simulink model "test_pmdc_speed_control"  (R2023a)
settings: Solver=FixedStepAuto  StartTime=0.0  StopTime=2  FixedStep=1e-5  RelTol=1e-3
values from neighbouring files (symbols this model uses):
  J = 0.05    [dcmotor_parameter.m]    (also in parabtl.m; pmdc_parameter.m = 0.00252; testpara.m = 0.00252)
  Ki = Kp/Ti    [parabtl.m]    (also in pmdc_parameter.m)
  Kiv = Kpv/Tiv    [parabtl.m]    (also in pmdc_parameter.m)
  Kp = (Ra*Ta*OmegaN)/(2*Zeta)    [parabtl.m]    (also in pmdc_parameter.m)
  Kpv = TMech/(2*Teq)    [parabtl.m]    (also in pmdc_parameter.m)
  KT = KE    (= 1.17113806452)    [dcmotor_parameter.m]    (also in parabtl.m; pmdc_parameter.m = 0.424975; testpara.m = 0.424975)
  La = 5.2e-3    (= 0.0052)    [dcmotor_parameter.m]    (also in parabtl.m; pmdc_parameter.m = 0.0017; testpara.m = 0.0017)
  Ra = 0.32    [dcmotor_parameter.m]    (also in parabtl.m; pmdc_parameter.m = 0.26; testpara.m = 0.26)
  Tfi = 1/(5*fsw)    (= 4e-05)    [parabtl.m]    (also in pmdc_parameter.m)
  Tfv = 5*Tfi    (= 0.0002)    [parabtl.m]    (also in pmdc_parameter.m)
  UaN = 400    [parabtl.m]    (also in pmdc_parameter.m = 140; testpara.m = 140)
libraries: spsMosfetLib x16, spsVoltageMeasurementLib x5, spsDCMachineLib x4, spsDCVoltageSourceLib x4, simulink x4, spsControlledVoltageSourceLib x1, sps_lib x1
settings Model: Creator=luand  LastModifiedBy=luand

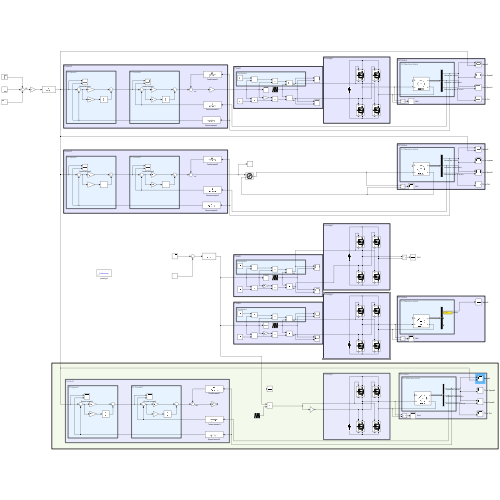
[thumbnail: Simulink's stored preview of the top-level diagram]
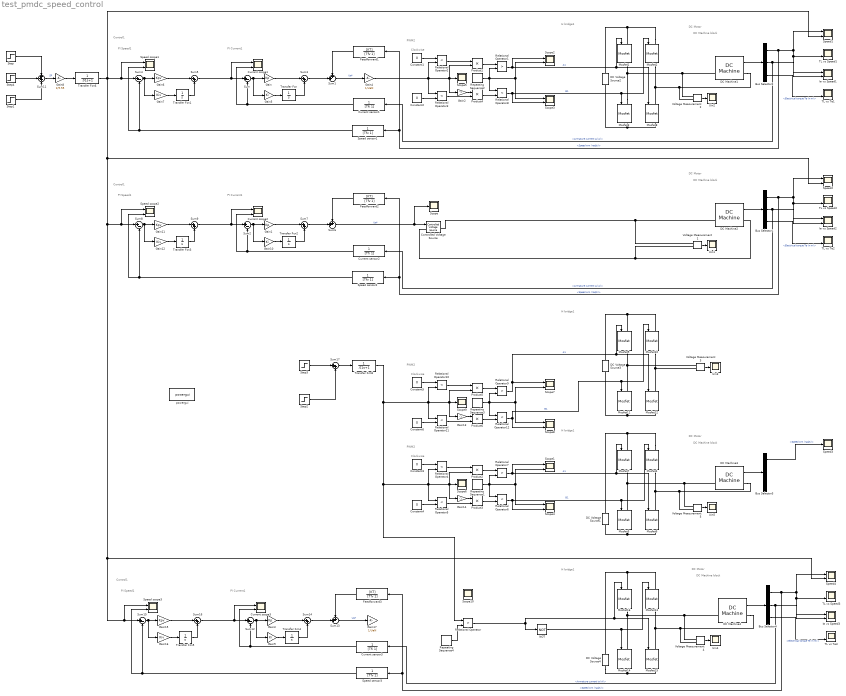
== system test_pmdc_speed_control ==
  note: PI Speed1
  note: PI Current1
  note: H bridge1
  note: PWM2
  note: Control1
  note: DC Motor
  note: DC Machine block
  note: Clockwise
  note: PI Speed1
  note: PI Current1
  note: Control1
  note: DC Motor
  note: DC Machine block
  note: H bridge1
  note: PWM2
  note: Clockwise
  note: H bridge1
  note: PWM2
  note: Clockwise
  note: DC Motor
  note: DC Machine block
  note: PI Speed1
  note: PI Current1
  note: Control1
  note: DC Motor
  note: DC Machine block
  note: H bridge1
  Bus Selector{1..4} (4 alike) : BusSelector  OutputSignals=Speed wm (rad/s),Armature current ia (A),Electrical torque Te (n m)
  Constant{1..6} (6 alike) : Constant  Value=0
  Controlled Voltage Source : spsControlledVoltageSourceLib/Controlled Voltage Source  Initialize=on  Source_Type=DC  Amplitude=0  Phase=0  Frequency=0  Measurements=None
  Current scope1 : Scope  NumInputPorts=2
  Current scope2 : Scope  NumInputPorts=2
  Current scope3 : Scope  NumInputPorts=2
  Current sensor1 : TransferFcn  Denominator=[Tfi 1]
  Current sensor2 : TransferFcn  Denominator=[Tfi 1]
  Current sensor3 : TransferFcn  Denominator=[Tfi 1]
  DC Machine{1..4} (4 alike) : spsDCMachineLib/DC Machine  PresetModel=No  MechanicalLoad=Torque TL  FieldType=Permanent magnet  ShowDetailedParameters=on  MeasurementBus=off  RLa=[ Ra La ]  RLf="[ 240  120]"  Laf=1.8  MachineConstant=Torque constant (N.m/A)  Ke=1.8  Kt=KT  J=J  Bm=0  Tf=0  w0=0  Ifinit=1  TsPowergui=0  TsBlock=-1
  DC Voltage Source{1..4} (4 alike) : spsDCVoltageSourceLib/DC Voltage Source  Amplitude=UaN  Measurements=None
  Feedforward1 : TransferFcn  Numerator=[KT]  Denominator=[Tfv 1]
  Feedforward2 : TransferFcn  Numerator=[KT]  Denominator=[Tfv 1]
  Feedforward3 : TransferFcn  Numerator=[KT]  Denominator=[Tfv 1]
  Gain : Gain  Gain=Kp
  Gain1 : Gain  Gain=Kp
  Gain10 : Gain  Gain=Ki
  Gain11 : Gain  Gain=Kpv
  Gain12 : Gain  Gain=Kiv
  Gain13 : Gain  Gain=-1
  Gain14 : Gain  Gain=-1
  Gain15 : Gain  Gain=Kpv
  Gain16 : Gain  Gain=Kiv
  Gain17 : Gain  Gain=1/UaN
  Gain2 : Gain  Gain=-1
  Gain3 : Gain  Gain=Kp
  Gain4 : Gain  Gain=1/UaN
  Gain5 : Gain  Gain=Ki
  Gain6 : Gain  Gain=Kpv
  Gain7 : Gain  Gain=Kiv
  Gain8 : Gain  Gain=1/9.55
  Gain9 : Gain  Gain=Ki
  Ia vs Speed1 : Scope  NumInputPorts=2
  Ia vs Speed2 : Scope  NumInputPorts=2
  Ia vs Speed3 : Scope  NumInputPorts=2
  Mosfet{1..3,8} (4 alike) : spsMosfetLib/Mosfet  Ron=0.1  Lon=0  Rd=0.01  Vfd=0  IC=0  Rs=1e5  Cs=inf  Measurements=on
  Mosfet{4..7,9..16} (12 alike) : spsMosfetLib/Mosfet  Ron=1e-3  Lon=0  Rd=0.01  Vfd=0  IC=0  Rs=1e5  Cs=inf  Measurements=on
  NOT : Logic  Operator=NOT  IconShape=distinctive  AllPortsSameDT=off  OutDataTypeStr=boolean
  Product{1..6} (6 alike) : Product
  Relational Operator{,1,7,9} (4 alike) : RelationalOperator  Operator=>  OutDataTypeStr=boolean  RndMeth=Simplest  InputSameDT=off
  Relational Operator{2..6,8,10..12} (9 alike) : RelationalOperator  Operator=<  OutDataTypeStr=boolean  RndMeth=Simplest  InputSameDT=off
  Repeating Sequence1 : simulink/Sources/Repeating Sequence  rep_seq_t=[0 1e-3]  rep_seq_y=[0 1]
  Repeating Sequence2 : simulink/Sources/Repeating Sequence  rep_seq_t=[0 1e-3]  rep_seq_y=[0 1]
  Repeating Sequence3 : simulink/Sources/Repeating Sequence  rep_seq_t=[0 1e-3]  rep_seq_y=[0 1]
  Repeating Sequence4 : simulink/Sources/Repeating Sequence  rep_seq_t=[0 5e-4 1e-3]  rep_seq_y=[-1 1 -1]
  Scope{,5..6,9..10} (5 alike) : Scope
  Scope{1..4,7..8} (6 alike) : Scope  NumInputPorts=2
  Speed scope1 : Scope  NumInputPorts=2
  Speed scope2 : Scope  NumInputPorts=2
  Speed scope3 : Scope  NumInputPorts=2
  Speed sensor1 : TransferFcn  Denominator=[Tfv 1]
  Speed sensor2 : TransferFcn  Denominator=[Tfv 1]
  Speed sensor3 : TransferFcn  Denominator=[Tfv 1]
  Speed1 : Scope  NumInputPorts=2
  Speed2 : Scope  NumInputPorts=2
  Speed3 : Scope
  Speed4 : Scope  NumInputPorts=2
  Step : Step  Time=0  After=3000  SampleTime=0
  Step1 : Step  Time=2  After=-1500  SampleTime=0
  Step2 : Step  After=-1  SampleTime=0
  Step3 : Step  Time=0  After=.5  SampleTime=0
  Step4 : Step  After=-1500  SampleTime=0
  Sum{,2,4,8,12,15} (6 alike) : Sum  Inputs=|+-
  Sum1 : Sum  Inputs=++|
  Sum11 : Sum  Inputs=+++
  Sum13 : Sum  Inputs=++|
  Sum{3,5,7,9,14,16..17} (7 alike) : Sum  Inputs=|++
  Sum6 : Sum  Inputs=++|
  TL vs Speed1 : Scope  NumInputPorts=2
  TL vs Speed2 : Scope  NumInputPorts=2
  TL vs Speed3 : Scope  NumInputPorts=2
  TL vs Te1 : Scope  NumInputPorts=2
  TL vs Te2 : Scope  NumInputPorts=2
  TL vs Te3 : Scope  NumInputPorts=2
  Transfer Fcn{,1..5} (6 alike) : TransferFcn  Denominator=[1 0]
  Transfer Fcn6 : TransferFcn  Denominator=[.01 1]
  Transfer Fcn8 : TransferFcn  Denominator=[.01 1]
  Uin{1..5} (5 alike) : Scope
  Voltage Measurement{1..5} (5 alike) : spsVoltageMeasurementLib/Voltage Measurement  PhasorSimulation=off  OutputType=Complex  PSBequivalent=0
  powergui : sps_lib/powergui  Priority=1  SimulationMode=Continuous  SampleTime=1e-5  frequency=60  Iterations=50  frequencyindice=0  Pbase=100e6  ErrMax=1e-4  UnitsV=kV  UnitsW=MW  buscounter=0  FunctionMessages=off  echomessages=off  EnableUseOfTLC=off  CurrentSourceSwitches=off  DisableSnubberDevices=off  DisableRonSwitches=off  DisableVfSwitches=off  DisplayEquations=off  AutomaticDiscreteSolvers=off  SolverType=Tustin/Backward Euler (TBE)  Interpol=off  ExternalGateDelay=off  methode=off  Ts=100  x0status=blocks  SPID=on  SwTol=0  HookPort=off  NonlinearTolerance=1e-4  nMaxIteration=100  ContinueOnMaxIteration=off  RestoreLinks=warning  ResistiveCurrentMeasurement=off  Frange=[0:2:500]  Ylog=off  Xlog=on  ShowGrid=off  save=off  variable=ZData  structure=0  ZoomFFT=off  StartTime=0.0  cycles=1  DisplayStyle=1  fundamental=60  FreqAxis=off  MaxFrequency=1000  frequencyindicesteady=1  RmsSteady=1  display=off
  wires:
  Sum11/1 -> Gain8/1  "SP"
  Relational Operator3/1 -> Product4/2
  Repeating Sequence2/1 -> Relational Operator1/2, Relational Operator8/1, Scope2/2, Scope3/1
  Gain4/1 -> Relational Operator3/1, Product1/2, Gain2/1, Scope5/1, Relational Operator2/2
  Relational Operator2/1 -> Product1/1
  Constant2/1 -> Relational Operator3/2
  Product4/1 -> Relational Operator8/2
  Gain2/1 -> Product4/1
  Constant1/1 -> Relational Operator2/1
  Relational Operator8/1 -> Mosfet2/1, Mosfet3/1, Scope3/2  "B1"
  Relational Operator1/1 -> Mosfet8/1, Mosfet1/1, Scope2/1  "A1"
  Product1/1 -> Relational Operator1/1
  Sum3/1 -> Sum1/2
  Bus Selector2/3 -> TL vs Te1/2  "<Electrical torque Te (n m)>"
  Bus Selector2/1 -> Feedforward1/1, Speed sensor1/1, Ia vs Speed1/2, TL vs Speed1/2, Speed1/1  "<Speed wm (rad/s)>"
  Bus Selector2/2 -> Ia vs Speed1/1, Current sensor1/1  "<Armature current ia (A)>"
  Voltage Measurement2/1 -> Uin2/1
  DC Machine1/1 -> Bus Selector2/1
  Sum5/1 -> Current scope1/1, Sum/1
  Current sensor1/1 -> Current scope1/2, Sum/2
  Sum/1 -> Gain5/1, Gain/1
  Gain5/1 -> Transfer Fcn/1
  Gain/1 -> Sum3/1
  Transfer Fcn/1 -> Sum3/2
  Transfer Fcn1/1 -> Sum5/2
  Gain6/1 -> Sum5/1
  Gain7/1 -> Transfer Fcn1/1
  Sum4/1 -> Gain7/1, Gain6/1
  Speed sensor1/1 -> Speed scope1/2, Sum4/2
  Sum1/1 -> Gain4/1  "Ua*"
  Feedforward1/1 -> Sum1/1
  Feedforward2/1 -> Sum6/1
  Sum6/1 -> Scope/1, Controlled Voltage Source/1  "Ua*"
  Speed sensor2/1 -> Sum8/2, Speed scope2/2
  Sum8/1 -> Gain11/1, Gain12/1
  Gain12/1 -> Transfer Fcn3/1
  Gain11/1 -> Sum9/1
  Transfer Fcn3/1 -> Sum9/2
  Transfer Fcn2/1 -> Sum7/2
  Gain1/1 -> Sum7/1
  Gain10/1 -> Transfer Fcn2/1
  Sum2/1 -> Gain1/1, Gain10/1
  Current sensor2/1 -> Sum2/2, Current scope2/2
  DC Machine2/1 -> Bus Selector1/1
  Voltage Measurement1/1 -> Uin1/1
  Bus Selector1/2 -> Current sensor2/1, Ia vs Speed2/1  "<Armature current ia (A)>"
  Bus Selector1/1 -> Speed2/1, TL vs Speed2/2, Ia vs Speed2/2, Speed sensor2/1, Feedforward2/1  "<Speed wm (rad/s)>"
  Bus Selector1/3 -> TL vs Te2/2  "<Electrical torque Te (n m)>"
  Sum7/1 -> Sum6/2
  Relational Operator11/1 -> Product6/2
  Repeating Sequence3/1 -> Relational Operator9/2, Relational Operator12/1, Scope7/2, Scope8/1
  Relational Operator10/1 -> Product5/1
  Constant6/1 -> Relational Operator11/2
  Product6/1 -> Relational Operator12/2
  Gain13/1 -> Product6/1
  Constant5/1 -> Relational Operator10/1
  Relational Operator12/1 -> Scope8/2, Mosfet11/1, Mosfet10/1  "B1"
  Relational Operator9/1 -> Scope7/1, Mosfet9/1, Mosfet12/1  "A1"
  Product5/1 -> Relational Operator9/1
  Voltage Measurement3/1 -> Uin3/1
  Product2/1 -> Relational Operator7/1
  Relational Operator7/1 -> Mosfet6/1, Mosfet7/1, Scope1/1  "A1"
  Relational Operator6/1 -> Mosfet5/1, Mosfet4/1, Scope4/2  "B1"
  Constant3/1 -> Relational Operator4/1
  Gain14/1 -> Product3/1
  Product3/1 -> Relational Operator6/2
  Constant4/1 -> Relational Operator5/2
  Relational Operator4/1 -> Product2/1
  Repeating Sequence1/1 -> Scope4/1, Scope1/2, Relational Operator6/1, Relational Operator7/2
  Relational Operator5/1 -> Product3/2
  Voltage Measurement5/1 -> Uin5/1
  DC Machine3/1 -> Bus Selector3/1
  Step3/1 -> Sum17/1
  Step/1 -> Sum11/1
  Step1/1 -> Sum11/3
  Sum14/1 -> Sum13/2
  Bus Selector4/3 -> TL vs Te3/2  "<Electrical torque Te (n m)>"
  Bus Selector4/1 -> Feedforward3/1, Speed sensor3/1, Ia vs Speed3/2, TL vs Speed3/2, Speed4/1  "<Speed wm (rad/s)>"
  Bus Selector4/2 -> Ia vs Speed3/1, Current sensor3/1  "<Armature current ia (A)>"
  Voltage Measurement4/1 -> Uin4/1
  DC Machine4/1 -> Bus Selector4/1
  Sum16/1 -> Current scope3/1, Sum12/1
  Current sensor3/1 -> Current scope3/2, Sum12/2
  Sum12/1 -> Gain9/1, Gain3/1
  Gain9/1 -> Transfer Fcn4/1
  Gain3/1 -> Sum14/1
  Transfer Fcn4/1 -> Sum14/2
  Transfer Fcn5/1 -> Sum16/2
  Gain15/1 -> Sum16/1
  Gain16/1 -> Transfer Fcn5/1
  Sum15/1 -> Gain16/1, Gain15/1
  Speed sensor3/1 -> Speed scope3/2, Sum15/2
  Gain8/1 -> Transfer Fcn6/1
  Sum13/1 -> Gain17/1  "Ua*"
  Feedforward3/1 -> Sum13/1
  NOT/1 -> Mosfet14/1, Mosfet13/1
  Repeating Sequence4/1 -> Relational Operator/2
  Relational Operator/1 -> NOT/1, Mosfet15/1, Mosfet16/1
  Transfer Fcn6/1 -> Speed1/2, Speed scope3/1, Sum15/1, Speed4/2, Sum8/1, Speed scope2/1, Speed2/2, Speed scope1/1, Sum4/1
  Sum17/1 -> Transfer Fcn8/1
  Bus Selector3/1 -> Speed3/1  "<Speed wm (rad/s)>"
  Step2/1 -> Sum17/2
  Sum9/1 -> Sum2/1, Current scope2/1
  Transfer Fcn8/1 -> Relational Operator/1, Relational Operator4/2, Scope6/1, Gain14/1, Product2/2, Relational Operator5/1, Relational Operator11/1, Product5/2, Gain13/1, Scope9/1, Relational Operator10/2
  Step4/1 -> Sum11/2
  connections:
  Voltage Measurement2/LConn2 -- DC Machine1/RConn1 -- Mosfet2/RConn1 -- Mosfet8/LConn1
  Mosfet3/LConn1 -- Mosfet1/RConn1 -- DC Machine1/LConn1 -- Voltage Measurement2/LConn1
  Mosfet2/LConn1 -- DC Voltage Source2/RConn1 -- Mosfet1/LConn1
  Mosfet3/RConn1 -- DC Voltage Source2/LConn1 -- Mosfet8/RConn1
  Voltage Measurement1/LConn2 -- DC Machine2/RConn1 -- Controlled Voltage Source/LConn1
  DC Machine2/LConn1 -- Controlled Voltage Source/RConn1 -- Voltage Measurement1/LConn1
  Mosfet10/RConn1 -- Mosfet12/LConn1 -- Voltage Measurement3/LConn2
  Mosfet9/RConn1 -- Voltage Measurement3/LConn1 -- Mosfet11/LConn1
  DC Voltage Source3/RConn1 -- Mosfet10/LConn1 -- Mosfet9/LConn1
  Mosfet11/RConn1 -- DC Voltage Source3/LConn1 -- Mosfet12/RConn1
  Mosfet4/RConn1 -- Voltage Measurement5/LConn2 -- DC Machine3/RConn1 -- Mosfet6/LConn1
  Mosfet7/RConn1 -- Voltage Measurement5/LConn1 -- DC Machine3/LConn1 -- Mosfet5/LConn1
  Mosfet4/LConn1 -- DC Voltage Source1/RConn1 -- Mosfet7/LConn1
  DC Voltage Source1/LConn1 -- Mosfet5/RConn1 -- Mosfet6/RConn1
  Mosfet16/LConn1 -- DC Voltage Source4/RConn1 -- Mosfet13/LConn1
  Mosfet14/RConn1 -- DC Voltage Source4/LConn1 -- Mosfet15/RConn1
  Mosfet14/LConn1 -- Mosfet16/RConn1 -- DC Machine4/LConn1 -- Voltage Measurement4/LConn1
  Voltage Measurement4/LConn2 -- Mosfet13/RConn1 -- Mosfet15/LConn1 -- DC Machine4/RConn1
